simulink model "double_esp32_udp"  (R2024b)
settings: Solver=FixedStepDiscrete  StartTime=0.0  StopTime=inf  FixedStep=0.01  RelTol=1e-3
libraries: dspnetwork x2
settings Model: Creator=Anny  LastModifiedBy=Anny

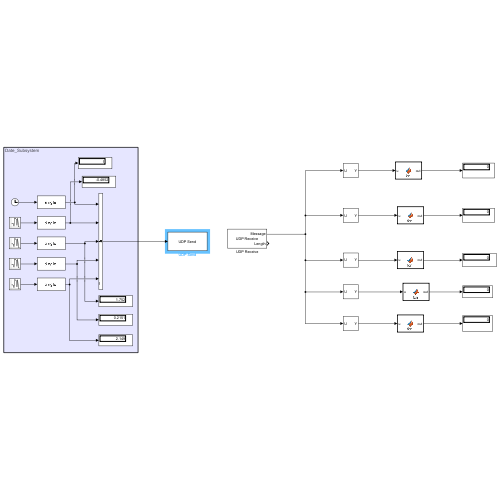
[thumbnail: Simulink's stored preview of the top-level diagram]
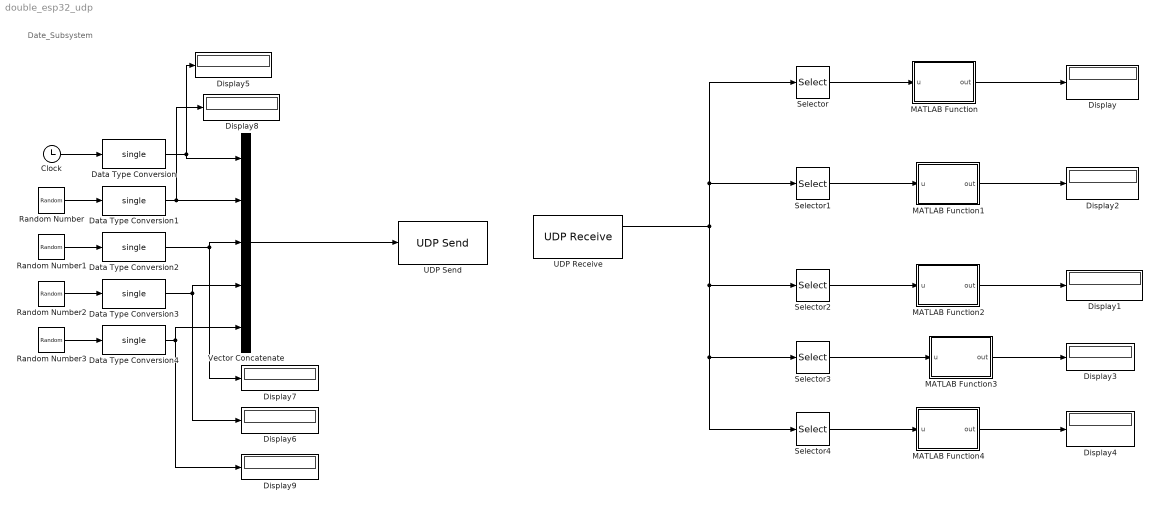
== system double_esp32_udp ==
  note: Date_Subsystem
  Clock : Clock
  Data Type Conversion{,1..4} (5 alike) : DataTypeConversion  OutDataTypeStr=single  SaturateOnIntegerOverflow=off  RndMeth=Floor
  Display{,1..9} (10 alike) : Display
  MATLAB Function : MATLAB Function  TreatAsAtomicUnit=on
  MATLAB Function1 : MATLAB Function  TreatAsAtomicUnit=on
  MATLAB Function2 : MATLAB Function  TreatAsAtomicUnit=on
  MATLAB Function3 : MATLAB Function  TreatAsAtomicUnit=on
  MATLAB Function4 : MATLAB Function  TreatAsAtomicUnit=on
  Random Number : RandomNumber  Seed=3  SampleTime=0.01
  Random Number1 : RandomNumber  Seed=4  SampleTime=.01
  Random Number2 : RandomNumber  Seed=5  SampleTime=0.01
  Random Number3 : RandomNumber  Seed=6  SampleTime=0.01
  Selector : Selector  InputPortWidth=20  IndexOptions=Index vector (dialog)  Indices=[1 2 3 4]  OutputSizes=1
  Selector1 : Selector  InputPortWidth=20  IndexOptions=Index vector (dialog)  Indices=[5 6 7 8]  OutputSizes=1
  Selector2 : Selector  InputPortWidth=20  IndexOptions=Index vector (dialog)  Indices=[9 10 11 12]  OutputSizes=1
  Selector3 : Selector  InputPortWidth=20  IndexOptions=Index vector (dialog)  Indices=[13 14 15 16]  OutputSizes=1
  Selector4 : Selector  InputPortWidth=20  IndexOptions=Index vector (dialog)  Indices=[17 18 19 20]  OutputSizes=1
  UDP Receive : dspnetwork/UDP Receive  localURL='0.0.0.0'  localPort=25001  remoteURL='0.0.0.0'  remotePort=-1  recvBufferSize=1024  dims=20  signalDatatype=uint8  isComplex=off  isVarSize=off  showBlockingTime=off  blockingTime=0  sampletime=0.01  blockPlatform=[]
      settings: LibrarySourceBlock=dspsrcs4/UDP Receive
  UDP Send : dspnetwork/UDP Send  remoteURL='172.20.10.2'  remotePort=12345  localURL='0.0.0.0'  localPortSource=Specify via dialog  localPort=25001  sendBufferSize=1024  sampletime=-1  blockPlatform=[]  separateLengthPort=0
      settings: LibrarySourceBlock=dspsnks4/UDP Send
  Vector Concatenate : Concatenate  NumInputs=5  Mode=Multidimensional array
  wires:
  Data Type Conversion/1 -> Vector Concatenate/1, Display5/1
  Data Type Conversion4/1 -> Vector Concatenate/5, Display9/1
  Random Number2/1 -> Data Type Conversion3/1
  Random Number3/1 -> Data Type Conversion4/1
  Data Type Conversion1/1 -> Vector Concatenate/2, Display8/1
  Random Number1/1 -> Data Type Conversion2/1
  Data Type Conversion3/1 -> Vector Concatenate/4, Display6/1
  Clock/1 -> Data Type Conversion/1
  Random Number/1 -> Data Type Conversion1/1
  Data Type Conversion2/1 -> Vector Concatenate/3, Display7/1
  Vector Concatenate/1 -> UDP Send/1
  MATLAB Function2/1(out) -> Display1/1
  Selector/1 -> MATLAB Function/1(u)
  Selector2/1 -> MATLAB Function2/1(u)
  Selector1/1 -> MATLAB Function1/1(u)
  Selector4/1 -> MATLAB Function4/1(u)
  MATLAB Function4/1(out) -> Display4/1
  UDP Receive/1 -> Selector4/1, Selector3/1, Selector2/1, Selector1/1, Selector/1
  MATLAB Function/1(out) -> Display/1
  MATLAB Function1/1(out) -> Display2/1
  Selector3/1 -> MATLAB Function3/1(u)
  MATLAB Function3/1(out) -> Display3/1

== matlab function double_esp32_udp/MATLAB Function ==
  data: u input uint8 size=[4 1]; out output single size=[1 1]
function out = fcn(u)
%#codegen
% u: [4x1] uint8
% out: single scalar

coder.varsize('out', [1 1], [0 0]); % 明确输出大小
out = typecast(uint8(u), 'single'); % 小端字节序转换
end

== matlab function double_esp32_udp/MATLAB Function2 ==
  data: u input uint8 size=[4 1]; out output single size=[1 1]
function out = fcn(u)
%#codegen
% u: [4x1] uint8
% out: single scalar

coder.varsize('out', [1 1], [0 0]); % 明确输出大小
out = typecast(uint8(u), 'single'); % 小端字节序转换
end

== matlab function double_esp32_udp/MATLAB Function3 ==
  data: u input uint8 size=[4 1]; out output single size=[1 1]
function out = fcn(u)
%#codegen
% u: [4x1] uint8
% out: single scalar

coder.varsize('out', [1 1], [0 0]); % 明确输出大小
out = typecast(uint8(u), 'single'); % 小端字节序转换
end

== matlab function double_esp32_udp/MATLAB Function4 ==
  data: u input uint8 size=[4 1]; out output single size=[1 1]
function out = fcn(u)
%#codegen
% u: [4x1] uint8
% out: single scalar

coder.varsize('out', [1 1], [0 0]); % 明确输出大小
out = typecast(uint8(u), 'single'); % 小端字节序转换
end

== matlab function double_esp32_udp/MATLAB Function1 ==
  data: u input uint8 size=[4 1]; out output single size=[1 1]
function out = fcn(u)
%#codegen
% u: [4x1] uint8
% out: single scalar

coder.varsize('out', [1 1], [0 0]); % 明确输出大小
out = typecast(uint8(u), 'single'); % 小端字节序转换
end
